simulink model "Microgrid_LCTLM_server"  (R2025b)
settings: Solver=ode3  StartTime=0.0  StopTime=1  FixedStep=params.sampleTime  RelTol=1e-3
InitFcn:
  | unitlmModelFile = get_param(bdroot, 'FileName');
  | if ~isempty(unitlmModelFile), addpath(fileparts(unitlmModelFile)); end
  | initialise_optimised_tlm_interface();
  | clear unitlmModelFile
StartFcn:
  | unitlmModelFile = get_param(bdroot, 'FileName'); if ~isempty(unitlmModelFile), addpath(fileparts(unitlmModelFile)); end; try, if exist('unitlm_timing_probe', 'file') == 2, unitlm_timing_probe('start', 'server', bdroot); else, warning('uniTLM:TimingProbeNotFound', 'unitlm_timing_probe.m not found on MATLAB path; timing probe disabled.'); end; catch unitlmTimingError, warning('uniTLM:TimingProbeFailed', 'unitlm_timing_probe failed: %s', unitlmTimingError.message); end; clear unitlmModelFile
StopFcn:
  | unitlmModelFile = get_param(bdroot, 'FileName'); if ~isempty(unitlmModelFile), addpath(fileparts(unitlmModelFile)); end; try, if exist('unitlm_timing_probe', 'file') == 2, unitlm_timing_probe('stop', 'server', bdroot); else, warning('uniTLM:TimingProbeNotFound', 'unitlm_timing_probe.m not found on MATLAB path; timing probe disabled.'); end; catch unitlmTimingError, warning('uniTLM:TimingProbeFailed', 'unitlm_timing_probe failed: %s', unitlmTimingError.message); end; clear unitlmModelFile
  | %% StopFcn: save TLM server-side results
  | 
  | modelName = bdroot;
  | modelFile = get_param(modelName, 'FileName');
  | 
  | if isempty(modelFile)
  |     modelDir = pwd;
  | else
  |     modelDir = fileparts(modelFile);
  | end
  | 
  | resultDir = fullfile(modelDir, 'result');
  | 
  | if ~exist(resultDir, 'dir')
  |     mkdir(resultDir);
  | end
  | 
  | % Server-side workspace variables
  | variableNames = {
  |     'server_voltage'
  |     'server_current'
  |     'server_PQ'
  | };
  | 
  | serverTLMData = struct();
  | 
  | for k = 1:numel(variableNames)
  | 
  |     originalName = variableNames{k};
  |     saveName = [originalName, '_TLM'];
  | 
  |     if evalin('base', sprintf('exist(''%s'', ''var'')', originalName))
  |         serverTLMData.(saveName) = evalin('base', originalName);
  |     else
  |         warning( ...
  |             'StopFcn:MissingVariable', ...
  |             'Variable "%s" was not found in the base workspace.', ...
  |             originalName);
  |     end
  | end
  | 
  | % Save to result/server_TLM.mat
  | saveFile = fullfile(resultDir, 'server_TLM.mat');
  | save(saveFile, '-struct', 'serverTLMData');
  | 
  | fprintf('TLM server-side results saved to:\n%s\n', saveFile);
values from neighbouring files (symbols this model uses):
  Cf = Cf_pu*Cb    [initialize_unitlm_microgrid.m]
  f = logspace(log10(fMin), log10(fMax), nFrequency).'    [fit_non_heaviside_line_rational.m]    (also in initialize_unitlm_microgrid.m = 50)
  fsw1 = 10e3    (= 10000)    [initialize_unitlm_microgrid.m]
  hr_lp_a = interface.hr_lp_a    [initialise_optimised_tlm_interface.m]
  hr_lp_b = interface.hr_lp_b    [initialise_optimised_tlm_interface.m]
  Ip = 2*P/(3*Vp)    [initialize_unitlm_microgrid.m]
  L1 = L1_pu*Lb    [initialize_unitlm_microgrid.m]
  L2 = L2_pu*Lb    [initialize_unitlm_microgrid.m]
  L3 = L3_pu*Lb    [initialize_unitlm_microgrid.m]
  L4 = L4_pu*Lb    [initialize_unitlm_microgrid.m]
  L_leakageinductance_1 = windingInductance(primaryWindingIndex)    [initialise_optimised_tlm_interface.m]
  L_magnetisation_1 = transformer.LmPu*primaryZbase/omegaNominal    [initialise_optimised_tlm_interface.m]
  L_remain_server = interface.L_remain_server    [initialise_optimised_tlm_interface.m]
  Lc = Lc_pu*Lb    [initialize_unitlm_microgrid.m]
  Lf2 = Lf2_pu*Lb    [initialize_unitlm_microgrid.m]
  line_aHr = interface.line_aHr    [initialise_optimised_tlm_interface.m]    (also in initialize_unitlm_microgrid.m = real(line_aHr))
  line_aZc = interface.line_aZc    [initialise_optimised_tlm_interface.m]    (also in initialize_unitlm_microgrid.m = real(line_aZc))
  line_bHr = interface.line_bHr    [initialise_optimised_tlm_interface.m]    (also in initialize_unitlm_microgrid.m = real(line_bHr))
  line_bZc = interface.line_bZc    [initialise_optimised_tlm_interface.m]    (also in initialize_unitlm_microgrid.m = real(line_bZc))
  P = 5e6    (= 5000000)    [initialize_unitlm_microgrid.m]
  params = varargin{1}    [Client_co.m]    (also in Client_co_TLM.m; Server_co.m; Server_co_TLM.m; initialise_optimised_tlm_interface.m = config.cosimParams)
  R1 = R1_pu*Zb    [initialize_unitlm_microgrid.m]
  R2 = R2_pu*Zb    [initialize_unitlm_microgrid.m]
  R3 = R3_pu*Zb    [initialize_unitlm_microgrid.m]
  R4 = R4_pu*Zb    [initialize_unitlm_microgrid.m]
  R_copperloss_1 = windingResistance(primaryWindingIndex)    [initialise_optimised_tlm_interface.m]
  R_coreloss_1 = transformer.RmPu*primaryZbase    [initialise_optimised_tlm_interface.m]
  R_remain_server = interface.R_remain_server    [initialise_optimised_tlm_interface.m]
  Rbreaker = Rbreaker_pu*Zb    [initialize_unitlm_microgrid.m]
  Rdamp = Rf    [initialize_unitlm_microgrid.m]
  Rf = Rf_pu*Zb    [initialize_unitlm_microgrid.m]
  Rload1 = Vp/Ip    [initialize_unitlm_microgrid.m]
  Rload2 = Vp/Ip    [initialize_unitlm_microgrid.m]
  Rload3 = Vp/Ip    [initialize_unitlm_microgrid.m]
  Rv_pu = 0.1    [initialize_unitlm_microgrid.m]
  Sxfmr = 6.3e6    (= 6300000)    [initialize_unitlm_microgrid.m]
  Vac = sqrt(2)*Vline/sqrt(3)    [initialize_unitlm_microgrid.m]
  Vhv = 66e3    (= 66000)    [initialize_unitlm_microgrid.m]
  Vline = 690    [initialize_unitlm_microgrid.m]
  Vp = Vac    [initialize_unitlm_microgrid.m]
  Wb = 2*pi*f    (= 314.159265359)    [initialize_unitlm_microgrid.m]
  Xv_pu = 0.3    [initialize_unitlm_microgrid.m]
  Zc_base_L = interface.Zc_base_L    [initialise_optimised_tlm_interface.m]
  Zc_base_R = interface.Zc_base_R    [initialise_optimised_tlm_interface.m]
undefined symbols (not defined in the file or in its folder): DiscIntNeverNeededParam, DPL, dspblkCoreblockFVToolHelper, gcbh, Lline1
libraries: spsThreePhaseSeriesRLCBranchLib x18, spsControlledVoltageSourceLib x12, spsThreePhaseVIMeasurementLib x7, spsabctodq0Lib x6, simulink x4, slpidlib x4, spsThreePhaseBreakerLib x4, SimplusGT x3, spsThreePhaseTransformerTwoWindingsLib x3, spsPower3phInstantaneousLib x2, spsdq0toabcLib x2, spsDistributedParametersLineLib x1
(part 3 of 4)

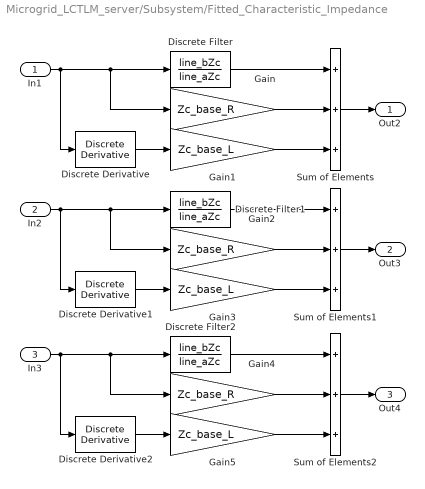
== system Microgrid_LCTLM_server/Subsystem/Fitted_Characteristic_Impedance ==
  In1 : Inport
  In2 : Inport  Port=2
  In3 : Inport  Port=3
  Discrete Derivative : simulink/Discrete/Discrete Derivative  gainval=1.0  ICPrevScaledInput=0.0  OutMin=[]  OutMax=[]  OutDataType=fixdt(1, 16)  OutScaling=2^-10  DoSatur=off
  Discrete Derivative1 : simulink/Discrete/Discrete Derivative  gainval=1.0  ICPrevScaledInput=0.0  OutMin=[]  OutMax=[]  OutDataType=fixdt(1, 16)  OutScaling=2^-10  DoSatur=off
  Discrete Derivative2 : simulink/Discrete/Discrete Derivative  gainval=1.0  ICPrevScaledInput=0.0  OutMin=[]  OutMax=[]  OutDataType=fixdt(1, 16)  OutScaling=2^-10  DoSatur=off
  Discrete Filter : DiscreteFilter  LoadFcn=dspblkCoreblockFVToolHelper(gcbh,'load');  Numerator=line_bZc  Denominator=line_aZc
      settings: CopyFcn=dspblkCoreblockFVToolHelper(gcbh,'copy');  DeleteFcn=dspblkCoreblockFVToolHelper(gcbh,'close');  ModelCloseFcn=dspblkCoreblockFVToolHelper(gcbh,'close');  PreSaveFcn=dspblkCoreblockFVToolHelper(gcbh,'presave');  PostSaveFcn=dspblkCoreblockFVToolHelper(gcbh,'postsave');  CloseFcn=dspblkCoreblockFVToolHelper(gcbh,'close');
  Discrete Filter1 : DiscreteFilter  LoadFcn=dspblkCoreblockFVToolHelper(gcbh,'load');  Numerator=line_bZc  Denominator=line_aZc
      settings: CopyFcn=dspblkCoreblockFVToolHelper(gcbh,'copy');  DeleteFcn=dspblkCoreblockFVToolHelper(gcbh,'close');  ModelCloseFcn=dspblkCoreblockFVToolHelper(gcbh,'close');  PreSaveFcn=dspblkCoreblockFVToolHelper(gcbh,'presave');  PostSaveFcn=dspblkCoreblockFVToolHelper(gcbh,'postsave');  CloseFcn=dspblkCoreblockFVToolHelper(gcbh,'close');
  Discrete Filter2 : DiscreteFilter  LoadFcn=dspblkCoreblockFVToolHelper(gcbh,'load');  Numerator=line_bZc  Denominator=line_aZc
      settings: CopyFcn=dspblkCoreblockFVToolHelper(gcbh,'copy');  DeleteFcn=dspblkCoreblockFVToolHelper(gcbh,'close');  ModelCloseFcn=dspblkCoreblockFVToolHelper(gcbh,'close');  PreSaveFcn=dspblkCoreblockFVToolHelper(gcbh,'presave');  PostSaveFcn=dspblkCoreblockFVToolHelper(gcbh,'postsave');  CloseFcn=dspblkCoreblockFVToolHelper(gcbh,'close');
  Gain : Gain  Gain=Zc_base_R
  Gain1 : Gain  Gain=Zc_base_L
  Gain2 : Gain  Gain=Zc_base_R
  Gain3 : Gain  Gain=Zc_base_L
  Gain4 : Gain  Gain=Zc_base_R
  Gain5 : Gain  Gain=Zc_base_L
  Sum of Elements : Sum  Inputs=+++
  Sum of Elements1 : Sum  Inputs=+++
  Sum of Elements2 : Sum  Inputs=+++
  Out2 : Outport
  Out3 : Outport  Port=2
  Out4 : Outport  Port=3
  wires:
  In1/1 -> Gain/1, Discrete Filter/1, Discrete Derivative/1
  Discrete Derivative/1 -> Gain1/1
  Gain/1 -> Sum of Elements/2
  Gain1/1 -> Sum of Elements/3
  Discrete Filter/1 -> Sum of Elements/1
  Sum of Elements/1 -> Out2/1
  Gain2/1 -> Sum of Elements1/2
  Discrete Filter1/1 -> Sum of Elements1/1
  Sum of Elements1/1 -> Out3/1
  Discrete Derivative1/1 -> Gain3/1
  Gain3/1 -> Sum of Elements1/3
  In2/1 -> Gain2/1, Discrete Filter1/1, Discrete Derivative1/1
  Gain5/1 -> Sum of Elements2/3
  Discrete Derivative2/1 -> Gain5/1
  Discrete Filter2/1 -> Sum of Elements2/1
  Gain4/1 -> Sum of Elements2/2
  Sum of Elements2/1 -> Out4/1
  In3/1 -> Gain4/1, Discrete Filter2/1, Discrete Derivative2/1

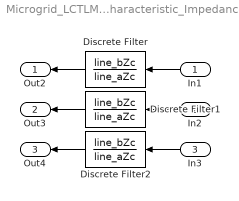
== system Microgrid_LCTLM_server/Subsystem/Fitted_Characteristic_Impedance1 ==
  In1 : Inport
  In2 : Inport  Port=2
  In3 : Inport  Port=3
  Discrete Filter : DiscreteFilter  LoadFcn=dspblkCoreblockFVToolHelper(gcbh,'load');  Numerator=line_bZc  Denominator=line_aZc
      settings: CopyFcn=dspblkCoreblockFVToolHelper(gcbh,'copy');  DeleteFcn=dspblkCoreblockFVToolHelper(gcbh,'close');  ModelCloseFcn=dspblkCoreblockFVToolHelper(gcbh,'close');  PreSaveFcn=dspblkCoreblockFVToolHelper(gcbh,'presave');  PostSaveFcn=dspblkCoreblockFVToolHelper(gcbh,'postsave');  CloseFcn=dspblkCoreblockFVToolHelper(gcbh,'close');
  Discrete Filter1 : DiscreteFilter  LoadFcn=dspblkCoreblockFVToolHelper(gcbh,'load');  Numerator=line_bZc  Denominator=line_aZc
      settings: CopyFcn=dspblkCoreblockFVToolHelper(gcbh,'copy');  DeleteFcn=dspblkCoreblockFVToolHelper(gcbh,'close');  ModelCloseFcn=dspblkCoreblockFVToolHelper(gcbh,'close');  PreSaveFcn=dspblkCoreblockFVToolHelper(gcbh,'presave');  PostSaveFcn=dspblkCoreblockFVToolHelper(gcbh,'postsave');  CloseFcn=dspblkCoreblockFVToolHelper(gcbh,'close');
  Discrete Filter2 : DiscreteFilter  LoadFcn=dspblkCoreblockFVToolHelper(gcbh,'load');  Numerator=line_bZc  Denominator=line_aZc
      settings: CopyFcn=dspblkCoreblockFVToolHelper(gcbh,'copy');  DeleteFcn=dspblkCoreblockFVToolHelper(gcbh,'close');  ModelCloseFcn=dspblkCoreblockFVToolHelper(gcbh,'close');  PreSaveFcn=dspblkCoreblockFVToolHelper(gcbh,'presave');  PostSaveFcn=dspblkCoreblockFVToolHelper(gcbh,'postsave');  CloseFcn=dspblkCoreblockFVToolHelper(gcbh,'close');
  Out2 : Outport
  Out3 : Outport  Port=2
  Out4 : Outport  Port=3
  wires:
  In1/1 -> Discrete Filter/1
  In2/1 -> Discrete Filter1/1
  Discrete Filter1/1 -> Out3/1
  Discrete Filter2/1 -> Out4/1
  In3/1 -> Discrete Filter2/1
  Discrete Filter/1 -> Out2/1

== system Microgrid_LCTLM_server/Subsystem/Grid1 ==
  Controlled Voltage Source1 : spsControlledVoltageSourceLib/Controlled Voltage Source  Initialize=on  Source_Type=AC  Amplitude=0  Phase=0  Frequency=0  Measurements=None
  Controlled Voltage Source2 : spsControlledVoltageSourceLib/Controlled Voltage Source  Initialize=on  Source_Type=AC  Amplitude=0  Phase=0  Frequency=0  Measurements=None
  Controlled Voltage Source6 : spsControlledVoltageSourceLib/Controlled Voltage Source  Initialize=on  Source_Type=AC  Amplitude=0  Phase=0  Frequency=0  Measurements=None
  Subsystem20 : Subsystem
  a : PMIOPort  Side=Left
  b : PMIOPort  Port=2  Side=Left
  c : PMIOPort  Port=3  Side=Left
  wires:
  Subsystem20/3(Ec) -> Controlled Voltage Source6/1
  Subsystem20/1(Ea) -> Controlled Voltage Source1/1
  Subsystem20/2(Eb) -> Controlled Voltage Source2/1
  connections:
  Controlled Voltage Source1/RConn1 -- a/RConn1
  Controlled Voltage Source6/RConn1 -- c/RConn1
  Controlled Voltage Source6/LConn1 -- Controlled Voltage Source2/LConn1 -- Controlled Voltage Source1/LConn1
  Controlled Voltage Source2/RConn1 -- b/RConn1

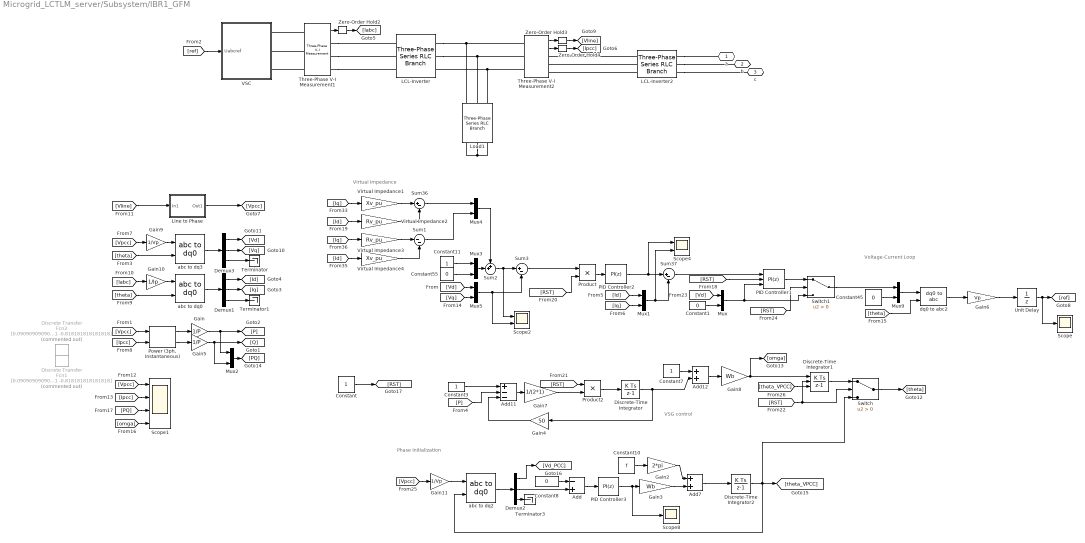
== system Microgrid_LCTLM_server/Subsystem/IBR1_GFM ==
  note: Voltage-Current Loop
  note: VSG control
  note: Virtual Impedance
  note: Phase Initialization
  Add : Sum  Inputs=-+
  Add11 : Sum  Inputs=+--
  Add12 : Sum
  Add7 : Sum
  Constant : Constant
  Constant{1,8,45,55} (4 alike) : Constant  Value=0
  Constant10 : Constant  Value=f
  Constant11 : Constant  SampleTime=-1
  Constant3 : Constant
  Constant7 : Constant
  Demux1 : Demux  Outputs=3
  Demux2 : Demux  Outputs=3
  Demux3 : Demux  Outputs=3
  Discrete Transfer Fcn1 : DiscreteTransferFcn  Commented=on  Numerator=[0.090909090909091 0.090909090909091]  Denominator=[1 -0.818181818181818]
  Discrete Transfer Fcn2 : DiscreteTransferFcn  Commented=on  Numerator=[0.090909090909091 0.090909090909091]  Denominator=[1 -0.818181818181818]
  Discrete-Time Integrator : DiscreteIntegrator  SampleTime=1/fsw1  ICPrevOutput=DiscIntNeverNeededParam  ICPrevScaledInput=DiscIntNeverNeededParam
  Discrete-Time Integrator1 : DiscreteIntegrator  ExternalReset=rising  InitialConditionSource=external  SampleTime=1/fsw1  ICPrevOutput=DiscIntNeverNeededParam  ICPrevScaledInput=DiscIntNeverNeededParam
  Discrete-Time Integrator2 : DiscreteIntegrator  SampleTime=1/fsw1  ICPrevOutput=DiscIntNeverNeededParam  ICPrevScaledInput=DiscIntNeverNeededParam
  Gain : Gain  Gain=1/P
  Gain10 : Gain  Gain=1/Ip
  Gain11 : Gain  Gain=1/Vp
  Gain2 : Gain  Gain=2*pi
  Gain3 : Gain  Gain=Wb
  Gain4 : Gain  Gain=50
  Gain5 : Gain  Gain=1/P
  Gain6 : Gain  Gain=Vp
  Gain7 : Gain  Gain=1/(2*1)
  Gain8 : Gain  Gain=Wb
  Gain9 : Gain  Gain=1/Vp
  LCL-Inverter : spsThreePhaseSeriesRLCBranchLib/Three-Phase Series RLC Branch  LConnTagsString=A|B|C  RConnTagsString=A|B|C  BranchType=RL  Resistance=Rf  Inductance=Lc  Capacitance=1e-6  Measurements=None
  LCL-Inverter2 : spsThreePhaseSeriesRLCBranchLib/Three-Phase Series RLC Branch  LConnTagsString=A|B|C  RConnTagsString=A|B|C  BranchType=RL  Resistance=Rf  Inductance=Lf2  Capacitance=1e-6  Measurements=None
  Line to Phase : Subsystem
  Load1 : spsThreePhaseSeriesRLCBranchLib/Three-Phase Series RLC Branch  LConnTagsString=A|B|C  RConnTagsString=A|B|C  BranchType=RC  Resistance=Rdamp  Inductance=1e-3  Capacitance=Cf  Measurements=None
  Mux{,1..5,9} (7 alike) : Mux  Inputs=2
  PID Controller1 : slpidlib/PID Controller  Controller=PI  Form=Parallel  TimeDomain=Discrete-time  UseExternalTs=off  SampleTime=1/fsw1  IntegratorMethod=Forward Euler  FilterMethod=Forward Euler  ControllerParametersSource=internal  P=0.5  I=100  UseKiTs=off  D=0  UseExternalDerivativeSource=off  N=100  UseFilter=on  TunerSelectOption=Transfer Function Based (PID Tuner App)  InitialConditionSource=external  InitialConditionForIntegrator=0  InitialConditionForFilter=0  DifferentiatorICPrevScaledInput=0  ExternalReset=rising  TrackingMode=off  Kt=1  LimitOutput=off  SatLimitsSource=internal  UpperSaturationLimit=inf  LowerSaturationLimit=-inf  LinearizeAsGain=on  AntiWindupMode=none  Kb=1  LimitIntegrator=off  UpperIntegratorSaturationLimit=inf  LowerIntegratorSaturationLimit=-inf  POutMin=[]  POutMax=[]  IOutMin=[]  IOutMax=[]  DOutMin=[]  DOutMax=[]  NOutMin=[]  NOutMax=[]  SumOutMin=[]  SumOutMax=[]  SaturationOutMin=[]  SaturationOutMax=[]  PParamMin=[]  PParamMax=[]  IParamMin=[]  IParamMax=[]  DParamMin=[]  DParamMax=[]  NParamMin=[]  NParamMax=[]  KbParamMin=[]  KbParamMax=[]  KtParamMin=[]  KtParamMax=[]  KbOutMin=[]  KbOutMax=[]  KtOutMin=[]  KtOutMax=[]  IntegratorOutMin=[]  IntegratorOutMax=[]  FilterOutMin=[]  FilterOutMax=[]  SumI1OutMin=[]  SumI1OutMax=[]  SumI2OutMin=[]  SumI2OutMax=[]  SumI3OutMin=[]  SumI3OutMax=[]  SumI4OutMin=[]  SumI4OutMax=[]  SumDOutMin=[]  SumDOutMax=[]  DifferentiatorOutMin=[]  DifferentiatorOutMax=[]  FilterDiffOutCoefMin=[]  FilterDiffOutCoefMax=[]  ReciprocalOutMin=[]  ReciprocalOutMax=[]  SumDenOutMin=[]  SumDenOutMax=[]  SumNumOutMin=[]  SumNumOutMax=[]  DivideOutMin=[]  DivideOutMax=[]  UdiffTsProdOutMin=[]  UdiffTsProdOutMax=[]  NTsProdOutMin=[]  NTsProdOutMax=[]  UintegralTsProdOutMin=[]  UintegralTsProdOutMax=[]  UngainTsProdOutMin=[]  UngainTsProdOutMax=[]  ClampingZeroOutDataTypeStr=Inherit: Inherit via back propagation  ClampingZeroOutMin=[]  ClampingZeroOutMax=[]  FilterDenConstantOutDataTypeStr=Inherit: Inherit via back propagation  FilterDenConstantOutMin=[]  FilterDenConstantOutMax=[]  PCopyOutDataTypeStr=Inherit: Inherit via back propagation  PCopyOutMin=[]  PCopyOutMax=[]  NCopyOutDataTypeStr=Inherit: Inherit via back propagation  NCopyOutMin=[]  NCopyOutMax=[]  IntegratorContinuousStateAttributes=''  IntegratorStateMustResolveToSignalObject=off  IntegratorRTWStateStorageClass=Auto  FilterContinuousStateAttributes=''  FilterStateMustResolveToSignalObject=off  FilterRTWStateStorageClass=Auto  ParallelPVariant=InternalParameters  IdealPVariant=Disabled  IVariant=InternalParameters  DVariant=Disabled  IntegratorVariant=Discrete  SatVariant=Disabled  AWVariant=Passthrough  PCopyVariant=Disabled  TRVariant=Disabled  FdbkBlocksVariant=Forward  IdealPFdbkVariant=Disabled  SatFdbkVariant=Disabled  DerivativeFilterVariant=Disabled  NVariant=Disabled  NCopyVariant=Disabled_SignalSpec  FilterICVariant=Disabled  IntegratorICVariant=ExternalICs  ExternalResetVariant=ExternalReset  TRSumVariant=Passthrough  SumFdbkVariant=Disabled  SumVariant=Sum_PI  TsampFilterVariant=InternalTs  TsampNgainVariant=Passthrough  TsampIntegralVariant=Disabled_SignalSpec  ExternalSaturationOutDataTypeStr=Inherit: Same as second input  DerivativeSourceVariant=Disabled  PreIntVariant=InternalPreInt
  PID Controller2 : slpidlib/PID Controller  Controller=PI  Form=Parallel  TimeDomain=Discrete-time  UseExternalTs=off  SampleTime=1/fsw1  IntegratorMethod=Forward Euler  FilterMethod=Forward Euler  ControllerParametersSource=internal  P=0.2  I=500  UseKiTs=off  D=0  UseExternalDerivativeSource=off  N=100  UseFilter=on  TunerSelectOption=Transfer Function Based (PID Tuner App)  InitialConditionSource=internal  InitialConditionForIntegrator=0  InitialConditionForFilter=0  DifferentiatorICPrevScaledInput=0  ExternalReset=none  TrackingMode=off  Kt=1  LimitOutput=off  SatLimitsSource=internal  UpperSaturationLimit=inf  LowerSaturationLimit=-inf  LinearizeAsGain=on  AntiWindupMode=none  Kb=1  LimitIntegrator=off  UpperIntegratorSaturationLimit=inf  LowerIntegratorSaturationLimit=-inf  POutMin=[]  POutMax=[]  IOutMin=[]  IOutMax=[]  DOutMin=[]  DOutMax=[]  NOutMin=[]  NOutMax=[]  SumOutMin=[]  SumOutMax=[]  SaturationOutMin=[]  SaturationOutMax=[]  PParamMin=[]  PParamMax=[]  IParamMin=[]  IParamMax=[]  DParamMin=[]  DParamMax=[]  NParamMin=[]  NParamMax=[]  KbParamMin=[]  KbParamMax=[]  KtParamMin=[]  KtParamMax=[]  KbOutMin=[]  KbOutMax=[]  KtOutMin=[]  KtOutMax=[]  IntegratorOutMin=[]  IntegratorOutMax=[]  FilterOutMin=[]  FilterOutMax=[]  SumI1OutMin=[]  SumI1OutMax=[]  SumI2OutMin=[]  SumI2OutMax=[]  SumI3OutMin=[]  SumI3OutMax=[]  SumI4OutMin=[]  SumI4OutMax=[]  SumDOutMin=[]  SumDOutMax=[]  DifferentiatorOutMin=[]  DifferentiatorOutMax=[]  FilterDiffOutCoefMin=[]  FilterDiffOutCoefMax=[]  ReciprocalOutMin=[]  ReciprocalOutMax=[]  SumDenOutMin=[]  SumDenOutMax=[]  SumNumOutMin=[]  SumNumOutMax=[]  DivideOutMin=[]  DivideOutMax=[]  UdiffTsProdOutMin=[]  UdiffTsProdOutMax=[]  NTsProdOutMin=[]  NTsProdOutMax=[]  UintegralTsProdOutMin=[]  UintegralTsProdOutMax=[]  UngainTsProdOutMin=[]  UngainTsProdOutMax=[]  ClampingZeroOutDataTypeStr=Inherit: Inherit via back propagation  ClampingZeroOutMin=[]  ClampingZeroOutMax=[]  FilterDenConstantOutDataTypeStr=Inherit: Inherit via back propagation  FilterDenConstantOutMin=[]  FilterDenConstantOutMax=[]  PCopyOutDataTypeStr=Inherit: Inherit via back propagation  PCopyOutMin=[]  PCopyOutMax=[]  NCopyOutDataTypeStr=Inherit: Inherit via back propagation  NCopyOutMin=[]  NCopyOutMax=[]  IntegratorContinuousStateAttributes=''  IntegratorStateMustResolveToSignalObject=off  IntegratorRTWStateStorageClass=Auto  FilterContinuousStateAttributes=''  FilterStateMustResolveToSignalObject=off  FilterRTWStateStorageClass=Auto  ParallelPVariant=InternalParameters  IdealPVariant=Disabled  IVariant=InternalParameters  DVariant=Disabled  IntegratorVariant=Discrete  SatVariant=Disabled  AWVariant=Passthrough  PCopyVariant=Disabled  TRVariant=Disabled  FdbkBlocksVariant=Forward  IdealPFdbkVariant=Disabled  SatFdbkVariant=Disabled  DerivativeFilterVariant=Disabled  NVariant=Disabled  NCopyVariant=Disabled_SignalSpec  FilterICVariant=Disabled  IntegratorICVariant=InternalICs  ExternalResetVariant=Disabled  TRSumVariant=Passthrough  SumFdbkVariant=Disabled  SumVariant=Sum_PI  TsampFilterVariant=InternalTs  TsampNgainVariant=Passthrough  TsampIntegralVariant=Disabled_SignalSpec  ExternalSaturationOutDataTypeStr=Inherit: Same as second input  DerivativeSourceVariant=Disabled  PreIntVariant=InternalPreInt
  PID Controller3 : slpidlib/PID Controller  Controller=PI  Form=Parallel  TimeDomain=Discrete-time  UseExternalTs=off  SampleTime=1/fsw1  IntegratorMethod=Forward Euler  FilterMethod=Forward Euler  ControllerParametersSource=internal  P=2  I=5  UseKiTs=off  D=0  UseExternalDerivativeSource=off  N=100  UseFilter=on  TunerSelectOption=Transfer Function Based (PID Tuner App)  InitialConditionSource=internal  InitialConditionForIntegrator=0  InitialConditionForFilter=0  DifferentiatorICPrevScaledInput=0  ExternalReset=none  TrackingMode=off  Kt=1  LimitOutput=off  SatLimitsSource=internal  UpperSaturationLimit=inf  LowerSaturationLimit=-inf  LinearizeAsGain=on  AntiWindupMode=none  Kb=1  LimitIntegrator=off  UpperIntegratorSaturationLimit=inf  LowerIntegratorSaturationLimit=-inf  POutMin=[]  POutMax=[]  IOutMin=[]  IOutMax=[]  DOutMin=[]  DOutMax=[]  NOutMin=[]  NOutMax=[]  SumOutMin=[]  SumOutMax=[]  SaturationOutMin=[]  SaturationOutMax=[]  PParamMin=[]  PParamMax=[]  IParamMin=[]  IParamMax=[]  DParamMin=[]  DParamMax=[]  NParamMin=[]  NParamMax=[]  KbParamMin=[]  KbParamMax=[]  KtParamMin=[]  KtParamMax=[]  KbOutMin=[]  KbOutMax=[]  KtOutMin=[]  KtOutMax=[]  IntegratorOutMin=[]  IntegratorOutMax=[]  FilterOutMin=[]  FilterOutMax=[]  SumI1OutMin=[]  SumI1OutMax=[]  SumI2OutMin=[]  SumI2OutMax=[]  SumI3OutMin=[]  SumI3OutMax=[]  SumI4OutMin=[]  SumI4OutMax=[]  SumDOutMin=[]  SumDOutMax=[]  DifferentiatorOutMin=[]  DifferentiatorOutMax=[]  FilterDiffOutCoefMin=[]  FilterDiffOutCoefMax=[]  ReciprocalOutMin=[]  ReciprocalOutMax=[]  SumDenOutMin=[]  SumDenOutMax=[]  SumNumOutMin=[]  SumNumOutMax=[]  DivideOutMin=[]  DivideOutMax=[]  UdiffTsProdOutMin=[]  UdiffTsProdOutMax=[]  NTsProdOutMin=[]  NTsProdOutMax=[]  UintegralTsProdOutMin=[]  UintegralTsProdOutMax=[]  UngainTsProdOutMin=[]  UngainTsProdOutMax=[]  ClampingZeroOutDataTypeStr=Inherit: Inherit via back propagation  ClampingZeroOutMin=[]  ClampingZeroOutMax=[]  FilterDenConstantOutDataTypeStr=Inherit: Inherit via back propagation  FilterDenConstantOutMin=[]  FilterDenConstantOutMax=[]  PCopyOutDataTypeStr=Inherit: Inherit via back propagation  PCopyOutMin=[]  PCopyOutMax=[]  NCopyOutDataTypeStr=Inherit: Inherit via back propagation  NCopyOutMin=[]  NCopyOutMax=[]  IntegratorContinuousStateAttributes=''  IntegratorStateMustResolveToSignalObject=off  IntegratorRTWStateStorageClass=Auto  FilterContinuousStateAttributes=''  FilterStateMustResolveToSignalObject=off  FilterRTWStateStorageClass=Auto  ParallelPVariant=InternalParameters  IdealPVariant=Disabled  IVariant=InternalParameters  DVariant=Disabled  IntegratorVariant=Discrete  SatVariant=Disabled  AWVariant=Passthrough  PCopyVariant=Disabled  TRVariant=Disabled  FdbkBlocksVariant=Forward  IdealPFdbkVariant=Disabled  SatFdbkVariant=Disabled  DerivativeFilterVariant=Disabled  NVariant=Disabled  NCopyVariant=Disabled_SignalSpec  FilterICVariant=Disabled  IntegratorICVariant=InternalICs  ExternalResetVariant=Disabled  TRSumVariant=Passthrough  SumFdbkVariant=Disabled  SumVariant=Sum_PI  TsampFilterVariant=InternalTs  TsampNgainVariant=Passthrough  TsampIntegralVariant=Disabled_SignalSpec  ExternalSaturationOutDataTypeStr=Inherit: Same as second input  DerivativeSourceVariant=Disabled  PreIntVariant=InternalPreInt
  "Power (3ph, Instantaneous)" : spsPower3phInstantaneousLib/Power (3ph, Instantaneous)
  Product : Product
  Product2 : Product
  Scope : Scope
      settings: ActiveDisplayYMinimum=-1487.20088  ActiveDisplayYMaximum=1156.37442  DataLoggingVariableName=ScopeData2
  Scope1 : Scope  NumInputPorts=4
      settings: ActiveDisplayYMinimum=-459.19644  ActiveDisplayYMaximum=463.11203  DataLoggingVariableName=ScopeData4
  Scope2 : Scope  NumInputPorts=2
      settings: ActiveDisplayYMinimum=-0.48353  ActiveDisplayYMaximum=1.26771
  Scope4 : Scope  NumInputPorts=2
      settings: ActiveDisplayYMinimum=-1.96338  ActiveDisplayYMaximum=2.79764  DataLoggingVariableName=ScopeData3
  Scope8 : Scope
      settings: ActiveDisplayYMinimum=-0.17841  ActiveDisplayYMaximum=0.07598  DataLoggingVariableName=ScopeData4
  Sum1 : Sum  Inputs=|--
  Sum2 : Sum  Inputs=++|
  Sum3 : Sum  Inputs=|+-
  Sum36 : Sum  Inputs=|+-
  Sum37 : Sum  Inputs=|+-
  Switch : Switch  Criteria=u2 > Threshold  SaturateOnIntegerOverflow=off  InputSameDT=off
  Switch1 : Switch  Criteria=u2 > Threshold  SaturateOnIntegerOverflow=off  InputSameDT=off
  Terminator : Terminator
  Terminator1 : Terminator
  Terminator3 : Terminator
  Three-Phase V-I Measurement1 : spsThreePhaseVIMeasurementLib/Three-Phase V-I Measurement  VoltageMeasurement=no  SetLabelV=off  LabelV=Vabc  Vpu=off  VpuLL=off  CurrentMeasurement=yes  SetLabelI=off  LabelI=Iabc  Ipu=off  Pbase=100e6  Vbase=500e3  OutputType=Complex  PhasorSimulation=off  PSBequivalent=0
  Three-Phase V-I Measurement2 : spsThreePhaseVIMeasurementLib/Three-Phase V-I Measurement  VoltageMeasurement=phase-to-phase  SetLabelV=off  LabelV=Vabc  Vpu=off  VpuLL=off  CurrentMeasurement=yes  SetLabelI=off  LabelI=Iabc  Ipu=off  Pbase=100e6  Vbase=500e3  OutputType=Complex  PhasorSimulation=off  PSBequivalent=0
  Unit Delay : UnitDelay  SampleTime=1/fsw1
  VSC : Subsystem
  Virtual Impedance1 : Gain  Gain=Xv_pu
  Virtual Impedance2 : Gain  Gain=Rv_pu
  Virtual Impedance3 : Gain  Gain=Rv_pu
  Virtual Impedance4 : Gain  Gain=Xv_pu
  Zero-Order Hold2 : ZeroOrderHold  SampleTime=1/fsw1
  Zero-Order Hold3 : ZeroOrderHold  SampleTime=1/fsw1
  Zero-Order Hold4 : ZeroOrderHold  SampleTime=1/fsw1
  abc to dq0 : spsabctodq0Lib/abc to dq0  Alignment=90 degrees behind phase A axis
  abc to dq2 : spsabctodq0Lib/abc to dq0  Alignment=90 degrees behind phase A axis
  abc to dq3 : spsabctodq0Lib/abc to dq0  Alignment=90 degrees behind phase A axis
  dq0 to abc2 : spsdq0toabcLib/dq0 to abc  Alignment=90 degrees behind phase A axis
  a : PMIOPort  Side=Right
  b : PMIOPort  Port=2  Side=Right
  c : PMIOPort  Port=3  Side=Right
  wires:
  Mux2/1 -> [PQ]
  [omga] -> Scope1/4
  [PQ] -> Scope1/3
  "Power (3ph, Instantaneous)"/1 -> Gain/1
  "Power (3ph, Instantaneous)"/2 -> Gain5/1
  [Ipcc] -> "Power (3ph, Instantaneous)"/2
  [Vpcc] -> "Power (3ph, Instantaneous)"/1
  [ref] -> VSC/1(Uabcref)
  Demux3/2 -> [Vq]
  Constant55/1 -> Mux3/2
  Mux9/1 -> dq0 to abc2/1
  [Vq] -> Mux5/2
  Add12/1 -> Gain8/1
  Constant3/1 -> Add11/1
  Mux3/1 -> Sum2/2
  Discrete-Time Integrator/1 -> Add12/2, Gain4/1
  Gain4/1 -> Add11/3
  [Vpcc] -> Gain9/1
  [Iq] -> Mux1/2
  Demux3/3 -> Terminator/1
  Constant45/1 -> Mux9/2
  Add11/1 -> Gain7/1
  [theta] -> abc to dq3/2
  [P] -> Add11/2
  dq0 to abc2/1 -> Gain6/1
  [Id] -> Mux1/1
  [theta] -> abc to dq0/2
  Unit Delay/1 -> Scope/1, [ref]
  Constant11/1 -> Mux3/1
  [Vd] -> Mux5/1
  PID Controller2/1 -> Scope4/1, Sum37/1
  Mux1/1 -> Scope4/2, Sum37/2
  Demux3/1 -> [Vd]
  Gain6/1 -> Unit Delay/1
  Gain10/1 -> abc to dq0/1
  Mux5/1 -> Sum3/2, Scope2/2
  abc to dq3/1 -> Demux3/1
  Constant7/1 -> Add12/1
  [theta] -> dq0 to abc2/2
  Three-Phase V-I Measurement1/1 -> Zero-Order Hold2/1
  Zero-Order Hold2/1 -> [Iabc]
  Three-Phase V-I Measurement2/2 -> Zero-Order Hold4/1
  Three-Phase V-I Measurement2/1 -> Zero-Order Hold3/1
  Zero-Order Hold3/1 -> [Vline]
  Zero-Order Hold4/1 -> [Ipcc]
  Gain9/1 -> abc to dq3/1
  [Iabc] -> Gain10/1
  abc to dq0/1 -> Demux1/1
  Demux1/1 -> [Id]
  Demux1/3 -> Terminator1/1
  Demux1/2 -> [Iq]
  [Vline] -> Line to Phase/1(In1)
  Line to Phase/1(Out1) -> [Vpcc]
  [Vpcc] -> Scope1/1
  [Ipcc] -> Scope1/2
  Gain/1 -> Mux2/1, [P]
  Gain5/1 -> Mux2/2, [Q]
  [Iq] -> Virtual Impedance3/1
  [Id] -> Virtual Impedance4/1
  [Id] -> Virtual Impedance2/1
  Sum36/1 -> Mux4/1
  [Iq] -> Virtual Impedance1/1
  Virtual Impedance1/1 -> Sum36/1
  Sum1/1 -> Mux4/2
  Virtual Impedance2/1 -> Sum36/2
  Virtual Impedance4/1 -> Sum1/2
  Virtual Impedance3/1 -> Sum1/1
  Mux4/1 -> Sum2/1
  [RST] -> Product/2
  Product/1 -> PID Controller2/1
  [RST] -> PID Controller1/2
  Gain7/1 -> Product2/2
  Product2/1 -> Discrete-Time Integrator/1
  [RST] -> Product2/1
  [RST] -> Switch/2, Discrete-Time Integrator1/2
  PID Controller3/1 -> Scope8/1, Gain3/1
  Constant8/1 -> Add/1
  abc to dq2/1 -> Demux2/1
  Demux2/2 -> Add/2
  Demux2/3 -> Terminator3/1
  [Vpcc] -> Gain11/1
  Constant10/1 -> Gain2/1
  Add/1 -> PID Controller3/1
  Gain2/1 -> Add7/1
  Gain3/1 -> Add7/2
  Discrete-Time Integrator2/1 -> Switch/3, [theta_VPCC], abc to dq2/2
  Gain11/1 -> abc to dq2/1
  Add7/1 -> Discrete-Time Integrator2/1
  Constant1/1 -> Mux/2
  [Vd] -> Mux/1
  Mux/1 -> Switch1/3, PID Controller1/3
  Constant/1 -> [RST]
  Gain8/1 -> Discrete-Time Integrator1/1, [omga]
  [theta_VPCC] -> Discrete-Time Integrator1/3
  Discrete-Time Integrator1/1 -> Switch/1
  Switch/1 -> [theta]
  PID Controller1/1 -> Switch1/1
  Switch1/1 -> Mux9/1
  [RST] -> Switch1/2
  Sum37/1 -> PID Controller1/1
  Sum2/1 -> Scope2/1, Sum3/1
  Sum3/1 -> Product/1
  Demux2/1 -> [Vd_PCC]
  connections:
  LCL-Inverter2/RConn1 -- a/RConn1
  Three-Phase V-I Measurement1/RConn1 -- LCL-Inverter/LConn1
  Load1/LConn2 -- LCL-Inverter/RConn2 -- Three-Phase V-I Measurement2/LConn2
  Load1/LConn3 -- LCL-Inverter/RConn3 -- Three-Phase V-I Measurement2/LConn3
  Load1/LConn1 -- LCL-Inverter/RConn1 -- Three-Phase V-I Measurement2/LConn1
  Three-Phase V-I Measurement1/RConn2 -- LCL-Inverter/LConn2
  Three-Phase V-I Measurement1/RConn3 -- LCL-Inverter/LConn3
  LCL-Inverter2/RConn2 -- b/RConn1
  LCL-Inverter2/LConn1 -- Three-Phase V-I Measurement2/RConn1
  LCL-Inverter2/RConn3 -- c/RConn1
  Load1/RConn3 -- Load1/RConn2 -- Load1/RConn1
  Three-Phase V-I Measurement1/LConn1 -- VSC/RConn1
  Three-Phase V-I Measurement1/LConn2 -- VSC/RConn2
  Three-Phase V-I Measurement1/LConn3 -- VSC/RConn3
  LCL-Inverter2/LConn2 -- Three-Phase V-I Measurement2/RConn2
  LCL-Inverter2/LConn3 -- Three-Phase V-I Measurement2/RConn3

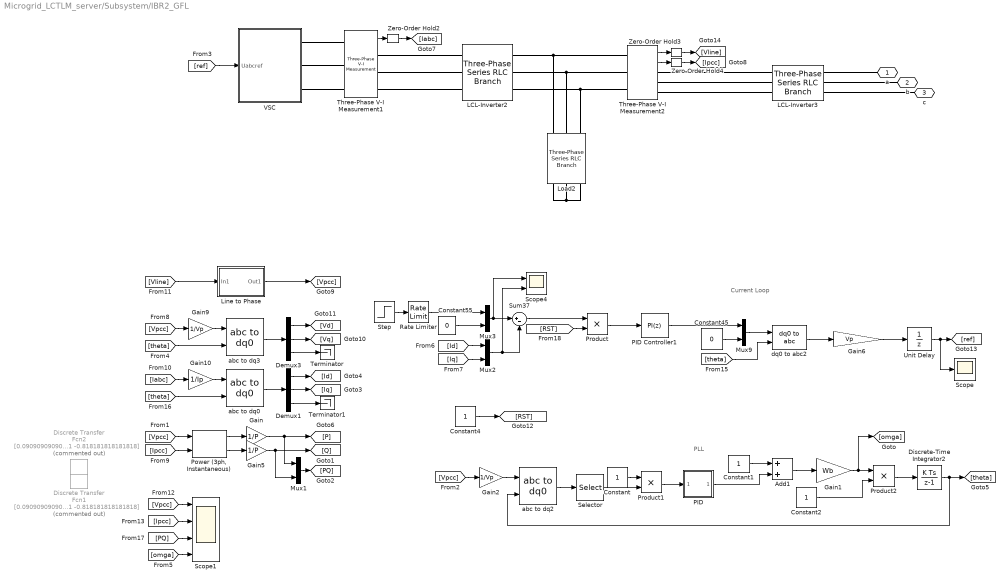
== system Microgrid_LCTLM_server/Subsystem/IBR2_GFL ==
  note: Current Loop
  note: PLL
  Add1 : Sum
  Constant{,1..2,4} (4 alike) : Constant
  Constant45 : Constant  Value=0
  Constant55 : Constant  Value=0
  Demux1 : Demux  Outputs=3
  Demux3 : Demux  Outputs=3
  Discrete Transfer Fcn1 : DiscreteTransferFcn  Commented=on  Numerator=[0.090909090909091 0.090909090909091]  Denominator=[1 -0.818181818181818]
  Discrete Transfer Fcn2 : DiscreteTransferFcn  Commented=on  Numerator=[0.090909090909091 0.090909090909091]  Denominator=[1 -0.818181818181818]
  Discrete-Time Integrator2 : DiscreteIntegrator  SampleTime=1/fsw1  ICPrevOutput=DiscIntNeverNeededParam  ICPrevScaledInput=DiscIntNeverNeededParam
  Gain : Gain  Gain=1/P
  Gain1 : Gain  Gain=Wb
  Gain10 : Gain  Gain=1/Ip
  Gain2 : Gain  Gain=1/Vp
  Gain5 : Gain  Gain=1/P
  Gain6 : Gain  Gain=Vp
  Gain9 : Gain  Gain=1/Vp
  LCL-Inverter2 : spsThreePhaseSeriesRLCBranchLib/Three-Phase Series RLC Branch  LConnTagsString=A|B|C  RConnTagsString=A|B|C  BranchType=RL  Resistance=Rf  Inductance=Lc  Capacitance=1e-6  Measurements=None
  LCL-Inverter3 : spsThreePhaseSeriesRLCBranchLib/Three-Phase Series RLC Branch  LConnTagsString=A|B|C  RConnTagsString=A|B|C  BranchType=RL  Resistance=Rf  Inductance=Lf2  Capacitance=1e-6  Measurements=None
  Line to Phase : Subsystem
  Load2 : spsThreePhaseSeriesRLCBranchLib/Three-Phase Series RLC Branch  LConnTagsString=A|B|C  RConnTagsString=A|B|C  BranchType=RC  Resistance=Rdamp  Inductance=1e-3  Capacitance=Cf  Measurements=None
  Mux{1..3,9} (4 alike) : Mux  Inputs=2
  PID : Subsystem
  PID Controller1 : slpidlib/PID Controller  Controller=PI  Form=Parallel  TimeDomain=Discrete-time  UseExternalTs=off  SampleTime=1/fsw1  IntegratorMethod=Forward Euler  FilterMethod=Forward Euler  ControllerParametersSource=internal  P=0.5  I=100  UseKiTs=off  D=0  UseExternalDerivativeSource=off  N=100  UseFilter=on  TunerSelectOption=Transfer Function Based (PID Tuner App)  InitialConditionSource=internal  InitialConditionForIntegrator=[1;0]  InitialConditionForFilter=0  DifferentiatorICPrevScaledInput=0  ExternalReset=none  TrackingMode=off  Kt=1  LimitOutput=off  SatLimitsSource=internal  UpperSaturationLimit=inf  LowerSaturationLimit=-inf  LinearizeAsGain=on  AntiWindupMode=none  Kb=1  LimitIntegrator=off  UpperIntegratorSaturationLimit=inf  LowerIntegratorSaturationLimit=-inf  POutMin=[]  POutMax=[]  IOutMin=[]  IOutMax=[]  DOutMin=[]  DOutMax=[]  NOutMin=[]  NOutMax=[]  SumOutMin=[]  SumOutMax=[]  SaturationOutMin=[]  SaturationOutMax=[]  PParamMin=[]  PParamMax=[]  IParamMin=[]  IParamMax=[]  DParamMin=[]  DParamMax=[]  NParamMin=[]  NParamMax=[]  KbParamMin=[]  KbParamMax=[]  KtParamMin=[]  KtParamMax=[]  KbOutMin=[]  KbOutMax=[]  KtOutMin=[]  KtOutMax=[]  IntegratorOutMin=[]  IntegratorOutMax=[]  FilterOutMin=[]  FilterOutMax=[]  SumI1OutMin=[]  SumI1OutMax=[]  SumI2OutMin=[]  SumI2OutMax=[]  SumI3OutMin=[]  SumI3OutMax=[]  SumI4OutMin=[]  SumI4OutMax=[]  SumDOutMin=[]  SumDOutMax=[]  DifferentiatorOutMin=[]  DifferentiatorOutMax=[]  FilterDiffOutCoefMin=[]  FilterDiffOutCoefMax=[]  ReciprocalOutMin=[]  ReciprocalOutMax=[]  SumDenOutMin=[]  SumDenOutMax=[]  SumNumOutMin=[]  SumNumOutMax=[]  DivideOutMin=[]  DivideOutMax=[]  UdiffTsProdOutMin=[]  UdiffTsProdOutMax=[]  NTsProdOutMin=[]  NTsProdOutMax=[]  UintegralTsProdOutMin=[]  UintegralTsProdOutMax=[]  UngainTsProdOutMin=[]  UngainTsProdOutMax=[]  ClampingZeroOutDataTypeStr=Inherit: Inherit via back propagation  ClampingZeroOutMin=[]  ClampingZeroOutMax=[]  FilterDenConstantOutDataTypeStr=Inherit: Inherit via back propagation  FilterDenConstantOutMin=[]  FilterDenConstantOutMax=[]  PCopyOutDataTypeStr=Inherit: Inherit via back propagation  PCopyOutMin=[]  PCopyOutMax=[]  NCopyOutDataTypeStr=Inherit: Inherit via back propagation  NCopyOutMin=[]  NCopyOutMax=[]  IntegratorContinuousStateAttributes=''  IntegratorStateMustResolveToSignalObject=off  IntegratorRTWStateStorageClass=Auto  FilterContinuousStateAttributes=''  FilterStateMustResolveToSignalObject=off  FilterRTWStateStorageClass=Auto  ParallelPVariant=InternalParameters  IdealPVariant=Disabled  IVariant=InternalParameters  DVariant=Disabled  IntegratorVariant=Discrete  SatVariant=Disabled  AWVariant=Passthrough  PCopyVariant=Disabled  TRVariant=Disabled  FdbkBlocksVariant=Forward  IdealPFdbkVariant=Disabled  SatFdbkVariant=Disabled  DerivativeFilterVariant=Disabled  NVariant=Disabled  NCopyVariant=Disabled_SignalSpec  FilterICVariant=Disabled  IntegratorICVariant=InternalICs  ExternalResetVariant=Disabled  TRSumVariant=Passthrough  SumFdbkVariant=Disabled  SumVariant=Sum_PI  TsampFilterVariant=InternalTs  TsampNgainVariant=Passthrough  TsampIntegralVariant=Disabled_SignalSpec  ExternalSaturationOutDataTypeStr=Inherit: Same as second input  DerivativeSourceVariant=Disabled  PreIntVariant=InternalPreInt
  "Power (3ph, Instantaneous)" : spsPower3phInstantaneousLib/Power (3ph, Instantaneous)
  Product : Product
  Product1 : Product
  Product2 : Product
  Rate Limiter : RateLimiter  RisingSlewLimit=5  FallingSlewLimit=-5  SampleTimeMode=inherited
  Scope : Scope
      settings: ActiveDisplayYMinimum=-423.55092  ActiveDisplayYMaximum=423.50002  DataLoggingVariableName=ScopeData3
  Scope1 : Scope  NumInputPorts=4
      settings: ActiveDisplayYMinimum=-435.11495  ActiveDisplayYMaximum=432.79484  DataLoggingVariableName=ScopeData5
  Scope4 : Scope  NumInputPorts=2
      settings: ActiveDisplayYMinimum=-1.88604  ActiveDisplayYMaximum=1.48102  DataLoggingVariableName=ScopeData8
  Selector : Selector  InputPortWidth=3  IndexOptions=Index vector (dialog)  Indices=[2]  OutputSizes=1
  Step : Step  Time=0  After=0.5  SampleTime=0
  Sum37 : Sum  Inputs=|+-
  Terminator : Terminator
  Terminator1 : Terminator
  Three-Phase V-I Measurement1 : spsThreePhaseVIMeasurementLib/Three-Phase V-I Measurement  VoltageMeasurement=no  SetLabelV=off  LabelV=Vabc  Vpu=off  VpuLL=off  CurrentMeasurement=yes  SetLabelI=off  LabelI=Iabc  Ipu=off  Pbase=100e6  Vbase=500e3  OutputType=Complex  PhasorSimulation=off  PSBequivalent=0
  Three-Phase V-I Measurement2 : spsThreePhaseVIMeasurementLib/Three-Phase V-I Measurement  VoltageMeasurement=phase-to-phase  SetLabelV=off  LabelV=Vabc  Vpu=off  VpuLL=off  CurrentMeasurement=yes  SetLabelI=off  LabelI=Iabc  Ipu=off  Pbase=100e6  Vbase=500e3  OutputType=Complex  PhasorSimulation=off  PSBequivalent=0
  Unit Delay : UnitDelay  SampleTime=1/fsw1
  VSC : Subsystem
  Zero-Order Hold2 : ZeroOrderHold  SampleTime=1/fsw1
  Zero-Order Hold3 : ZeroOrderHold  SampleTime=1/fsw1
  Zero-Order Hold4 : ZeroOrderHold  SampleTime=1/fsw1
  abc to dq0 : spsabctodq0Lib/abc to dq0  Alignment=90 degrees behind phase A axis
  abc to dq2 : spsabctodq0Lib/abc to dq0  Alignment=90 degrees behind phase A axis
  abc to dq3 : spsabctodq0Lib/abc to dq0  Alignment=90 degrees behind phase A axis
  dq0 to abc2 : spsdq0toabcLib/dq0 to abc  Alignment=90 degrees behind phase A axis
  a : PMIOPort  Side=Right
  b : PMIOPort  Port=2  Side=Right
  c : PMIOPort  Port=3  Side=Right
  wires:
  [Vpcc] -> Gain9/1
  Three-Phase V-I Measurement2/1 -> Zero-Order Hold3/1
  [Vline] -> Line to Phase/1(In1)
  Line to Phase/1(Out1) -> [Vpcc]
  Constant45/1 -> Mux9/2
  dq0 to abc2/1 -> Gain6/1
  Zero-Order Hold2/1 -> [Iabc]
  Three-Phase V-I Measurement1/1 -> Zero-Order Hold2/1
  Demux3/3 -> Terminator/1
  Zero-Order Hold4/1 -> [Ipcc]
  [theta] -> dq0 to abc2/2
  Demux1/2 -> [Iq]
  Gain6/1 -> Unit Delay/1
  abc to dq3/1 -> Demux3/1
  Demux3/1 -> [Vd]
  [Id] -> Mux2/1
  Mux2/1 -> Scope4/2, Sum37/2
  [Iq] -> Mux2/2
  Mux9/1 -> dq0 to abc2/1
  Constant55/1 -> Mux3/2
  [Iabc] -> Gain10/1
  Demux3/2 -> [Vq]
  Demux1/3 -> Terminator1/1
  Gain9/1 -> abc to dq3/1
  Demux1/1 -> [Id]
  Zero-Order Hold3/1 -> [Vline]
  Unit Delay/1 -> Scope/1, [ref]
  [ref] -> VSC/1(Uabcref)
  Three-Phase V-I Measurement2/2 -> Zero-Order Hold4/1
  Gain10/1 -> abc to dq0/1
  [theta] -> abc to dq3/2
  Mux3/1 -> Scope4/1, Sum37/1
  [theta] -> abc to dq0/2
  abc to dq0/1 -> Demux1/1
  Discrete-Time Integrator2/1 -> [theta], abc to dq2/2
  Constant1/1 -> Add1/1
  PID/1(Out1) -> Add1/2
  Add1/1 -> Gain1/1
  abc to dq2/1 -> Selector/1
  PID Controller1/1 -> Mux9/1
  Gain2/1 -> abc to dq2/1
  [Vpcc] -> Gain2/1
  "Power (3ph, Instantaneous)"/1 -> Gain/1
  "Power (3ph, Instantaneous)"/2 -> Gain5/1
  [Ipcc] -> "Power (3ph, Instantaneous)"/2
  [Vpcc] -> "Power (3ph, Instantaneous)"/1
  Gain/1 -> [P], Mux1/1
  [Vpcc] -> Scope1/1
  Gain5/1 -> [Q], Mux1/2
  [PQ] -> Scope1/3
  [Ipcc] -> Scope1/2
  [omga] -> Scope1/4
  Mux1/1 -> [PQ]
  Sum37/1 -> Product/1
  [RST] -> Product/2
  Product/1 -> PID Controller1/1
  Selector/1 -> Product1/2
  Product1/1 -> PID/1(In1)
  Product2/1 -> Discrete-Time Integrator2/1
  Gain1/1 -> [omga], Product2/1
  Constant/1 -> Product1/1
  Constant2/1 -> Product2/2
  Rate Limiter/1 -> Mux3/1
  Step/1 -> Rate Limiter/1
  Constant4/1 -> [RST]
  connections:
  Load2/RConn1 -- Load2/RConn3 -- Load2/RConn2
  LCL-Inverter2/RConn3 -- Load2/LConn3 -- Three-Phase V-I Measurement2/LConn3
  LCL-Inverter2/RConn2 -- Load2/LConn2 -- Three-Phase V-I Measurement2/LConn2
  LCL-Inverter2/RConn1 -- Load2/LConn1 -- Three-Phase V-I Measurement2/LConn1
  LCL-Inverter3/LConn2 -- Three-Phase V-I Measurement2/RConn2
  LCL-Inverter3/LConn3 -- Three-Phase V-I Measurement2/RConn3
  Three-Phase V-I Measurement1/LConn1 -- VSC/RConn1
  LCL-Inverter3/RConn3 -- c/RConn1
  Three-Phase V-I Measurement1/RConn3 -- LCL-Inverter2/LConn3
  Three-Phase V-I Measurement1/RConn2 -- LCL-Inverter2/LConn2
  Three-Phase V-I Measurement1/RConn1 -- LCL-Inverter2/LConn1
  Three-Phase V-I Measurement1/LConn2 -- VSC/RConn2
  LCL-Inverter3/RConn1 -- a/RConn1
  LCL-Inverter3/LConn1 -- Three-Phase V-I Measurement2/RConn1
  Three-Phase V-I Measurement1/LConn3 -- VSC/RConn3
  LCL-Inverter3/RConn2 -- b/RConn1

== system Microgrid_LCTLM_server/Subsystem/LOAD1 ==
  Constant8 : Constant  Value=0
  Rload1 : spsThreePhaseSeriesRLCBranchLib/Three-Phase Series RLC Branch  LConnTagsString=A|B|C  RConnTagsString=A|B|C  BranchType=R  Resistance=Rload1  Inductance=Lline1  Capacitance=1e-6  Measurements=None
  Three-Phase Breaker3 : spsThreePhaseBreakerLib/Three-Phase Breaker  InitialState=open  SwitchA=on  SwitchB=on  SwitchC=on  SwitchTimes=1.5  External=on  BreakerResistance=Rbreaker  SnubberResistance=1e6  SnubberCapacitance=inf  Measurements=None
  A : PMIOPort  Side=Left
  B : PMIOPort  Port=2  Side=Left
  C : PMIOPort  Port=3  Side=Left
  wires:
  Constant8/1 -> Three-Phase Breaker3/1
  connections:
  A/RConn1 -- Three-Phase Breaker3/LConn1
  Three-Phase Breaker3/RConn3 -- Rload1/LConn3
  B/RConn1 -- Three-Phase Breaker3/LConn2
  Rload1/RConn2 -- Rload1/RConn1 -- Rload1/RConn3
  Three-Phase Breaker3/RConn1 -- Rload1/LConn1
  Three-Phase Breaker3/RConn2 -- Rload1/LConn2
  C/RConn1 -- Three-Phase Breaker3/LConn3

== system Microgrid_LCTLM_server/Subsystem/LOAD3 ==
  Constant14 : Constant  Value=0
  Rload3 : spsThreePhaseSeriesRLCBranchLib/Three-Phase Series RLC Branch  LConnTagsString=A|B|C  RConnTagsString=A|B|C  BranchType=R  Resistance=Rload3  Inductance=Lline1  Capacitance=1e-6  Measurements=None
  Three-Phase Breaker2 : spsThreePhaseBreakerLib/Three-Phase Breaker  InitialState=open  SwitchA=on  SwitchB=on  SwitchC=on  SwitchTimes=1.5  External=on  BreakerResistance=Rbreaker  SnubberResistance=1e6  SnubberCapacitance=inf  Measurements=None
  A : PMIOPort  Side=Left
  B : PMIOPort  Port=2  Side=Left
  C : PMIOPort  Port=3  Side=Left
  wires:
  Constant14/1 -> Three-Phase Breaker2/1
  connections:
  Three-Phase Breaker2/LConn2 -- B/RConn1
  Three-Phase Breaker2/RConn1 -- Rload3/LConn1
  Three-Phase Breaker2/RConn3 -- Rload3/LConn3
  Rload3/RConn3 -- Rload3/RConn1 -- Rload3/RConn2
  Three-Phase Breaker2/RConn2 -- Rload3/LConn2
  Three-Phase Breaker2/LConn1 -- A/RConn1
  Three-Phase Breaker2/LConn3 -- C/RConn1

== system Microgrid_LCTLM_server/Subsystem/LOAD4 ==
  Constant1 : Constant
  Rload2 : spsThreePhaseSeriesRLCBranchLib/Three-Phase Series RLC Branch  LConnTagsString=A|B|C  RConnTagsString=A|B|C  BranchType=R  Resistance=Rload2  Inductance=Lline1  Capacitance=1e-6  Measurements=None
  Three-Phase Breaker1 : spsThreePhaseBreakerLib/Three-Phase Breaker  InitialState=open  SwitchA=on  SwitchB=on  SwitchC=on  SwitchTimes=1.5  External=on  BreakerResistance=Rbreaker  SnubberResistance=1e6  SnubberCapacitance=inf  Measurements=None
  A : PMIOPort  Side=Left
  B : PMIOPort  Port=2  Side=Left
  C : PMIOPort  Port=3  Side=Left
  wires:
  Constant1/1 -> Three-Phase Breaker1/1
  connections:
  Three-Phase Breaker1/RConn3 -- Rload2/LConn3
  B/RConn1 -- Three-Phase Breaker1/LConn2
  Three-Phase Breaker1/RConn1 -- Rload2/LConn1
  C/RConn1 -- Three-Phase Breaker1/LConn3
  Rload2/RConn3 -- Rload2/RConn2 -- Rload2/RConn1
  Three-Phase Breaker1/RConn2 -- Rload2/LConn2
  A/RConn1 -- Three-Phase Breaker1/LConn1

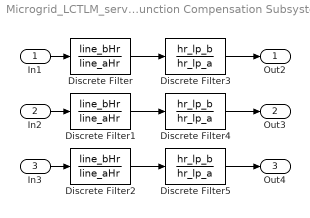
== system Microgrid_LCTLM_server/Subsystem/Propagation Function Compensation Subsystem ==
  In1 : Inport
  In2 : Inport  Port=2
  In3 : Inport  Port=3
  Discrete Filter : DiscreteFilter  LoadFcn=dspblkCoreblockFVToolHelper(gcbh,'load');  Numerator=line_bHr  Denominator=line_aHr
      settings: CopyFcn=dspblkCoreblockFVToolHelper(gcbh,'copy');  DeleteFcn=dspblkCoreblockFVToolHelper(gcbh,'close');  ModelCloseFcn=dspblkCoreblockFVToolHelper(gcbh,'close');  PreSaveFcn=dspblkCoreblockFVToolHelper(gcbh,'presave');  PostSaveFcn=dspblkCoreblockFVToolHelper(gcbh,'postsave');  CloseFcn=dspblkCoreblockFVToolHelper(gcbh,'close');
  Discrete Filter1 : DiscreteFilter  LoadFcn=dspblkCoreblockFVToolHelper(gcbh,'load');  Numerator=line_bHr  Denominator=line_aHr
      settings: CopyFcn=dspblkCoreblockFVToolHelper(gcbh,'copy');  DeleteFcn=dspblkCoreblockFVToolHelper(gcbh,'close');  ModelCloseFcn=dspblkCoreblockFVToolHelper(gcbh,'close');  PreSaveFcn=dspblkCoreblockFVToolHelper(gcbh,'presave');  PostSaveFcn=dspblkCoreblockFVToolHelper(gcbh,'postsave');  CloseFcn=dspblkCoreblockFVToolHelper(gcbh,'close');
  Discrete Filter2 : DiscreteFilter  LoadFcn=dspblkCoreblockFVToolHelper(gcbh,'load');  Numerator=line_bHr  Denominator=line_aHr
      settings: CopyFcn=dspblkCoreblockFVToolHelper(gcbh,'copy');  DeleteFcn=dspblkCoreblockFVToolHelper(gcbh,'close');  ModelCloseFcn=dspblkCoreblockFVToolHelper(gcbh,'close');  PreSaveFcn=dspblkCoreblockFVToolHelper(gcbh,'presave');  PostSaveFcn=dspblkCoreblockFVToolHelper(gcbh,'postsave');  CloseFcn=dspblkCoreblockFVToolHelper(gcbh,'close');
  Discrete Filter3 : DiscreteFilter  LoadFcn=dspblkCoreblockFVToolHelper(gcbh,'load');  Numerator=hr_lp_b  Denominator=hr_lp_a
      settings: CopyFcn=dspblkCoreblockFVToolHelper(gcbh,'copy');  DeleteFcn=dspblkCoreblockFVToolHelper(gcbh,'close');  ModelCloseFcn=dspblkCoreblockFVToolHelper(gcbh,'close');  PreSaveFcn=dspblkCoreblockFVToolHelper(gcbh,'presave');  PostSaveFcn=dspblkCoreblockFVToolHelper(gcbh,'postsave');  CloseFcn=dspblkCoreblockFVToolHelper(gcbh,'close');
  Discrete Filter4 : DiscreteFilter  LoadFcn=dspblkCoreblockFVToolHelper(gcbh,'load');  Numerator=hr_lp_b  Denominator=hr_lp_a
      settings: CopyFcn=dspblkCoreblockFVToolHelper(gcbh,'copy');  DeleteFcn=dspblkCoreblockFVToolHelper(gcbh,'close');  ModelCloseFcn=dspblkCoreblockFVToolHelper(gcbh,'close');  PreSaveFcn=dspblkCoreblockFVToolHelper(gcbh,'presave');  PostSaveFcn=dspblkCoreblockFVToolHelper(gcbh,'postsave');  CloseFcn=dspblkCoreblockFVToolHelper(gcbh,'close');
  Discrete Filter5 : DiscreteFilter  LoadFcn=dspblkCoreblockFVToolHelper(gcbh,'load');  Numerator=hr_lp_b  Denominator=hr_lp_a
      settings: CopyFcn=dspblkCoreblockFVToolHelper(gcbh,'copy');  DeleteFcn=dspblkCoreblockFVToolHelper(gcbh,'close');  ModelCloseFcn=dspblkCoreblockFVToolHelper(gcbh,'close');  PreSaveFcn=dspblkCoreblockFVToolHelper(gcbh,'presave');  PostSaveFcn=dspblkCoreblockFVToolHelper(gcbh,'postsave');  CloseFcn=dspblkCoreblockFVToolHelper(gcbh,'close');
  Out2 : Outport
  Out3 : Outport  Port=2
  Out4 : Outport  Port=3
  wires:
  In1/1 -> Discrete Filter/1
  In2/1 -> Discrete Filter1/1
  In3/1 -> Discrete Filter2/1
  Discrete Filter/1 -> Discrete Filter3/1
  Discrete Filter3/1 -> Out2/1
  Discrete Filter1/1 -> Discrete Filter4/1
  Discrete Filter4/1 -> Out3/1
  Discrete Filter5/1 -> Out4/1
  Discrete Filter2/1 -> Discrete Filter5/1

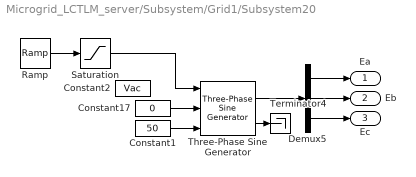
== system Microgrid_LCTLM_server/Subsystem/Grid1/Subsystem20 ==
  Constant1 : Constant  Value=50
  Constant17 : Constant  Value=0
  Constant2 : Constant  Value=Vac
  Demux5 : Demux  Outputs=3
  Ramp : simulink/Sources/Ramp  slope=Vac/0.01  start=0  InitialOutput=0
  Saturation : Saturate  UpperLimit=Vac  LowerLimit=0
  Terminator4 : Terminator
  Three-Phase Sine Generator : spsThreePhaseSineGeneratorLib/Three-Phase Sine Generator  Ts=1e-6
      settings: LibrarySourceBlock=|
      | sps_lib/Sources/Signal Generator Sources/Three-Phase
      | Sine Generator
  Ea : Outport
  Eb : Outport  Port=2
  Ec : Outport  Port=3
  wires:
  Three-Phase Sine Generator/1 -> Demux5/1
  Three-Phase Sine Generator/2 -> Terminator4/1
  Demux5/1 -> Ea/1
  Demux5/2 -> Eb/1
  Demux5/3 -> Ec/1
  Constant17/1 -> Three-Phase Sine Generator/2
  Constant1/1 -> Three-Phase Sine Generator/3
  Ramp/1 -> Saturation/1
  Saturation/1 -> Three-Phase Sine Generator/1

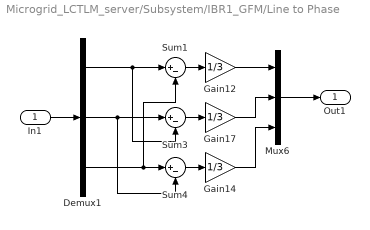
== system Microgrid_LCTLM_server/Subsystem/IBR1_GFM/Line to Phase ==
  In1 : Inport
  Demux1 : Demux  Outputs=3
  Gain12 : Gain  Gain=1/3
  Gain14 : Gain  Gain=1/3
  Gain17 : Gain  Gain=1/3
  Mux6 : Mux  Inputs=3
  Sum1 : Sum  Inputs=|+-
  Sum3 : Sum  Inputs=|+-
  Sum4 : Sum  Inputs=|+-
  Out1 : Outport
  wires:
  Sum3/1 -> Gain17/1
  Gain17/1 -> Mux6/2
  In1/1 -> Demux1/1
  Gain14/1 -> Mux6/3
  Sum1/1 -> Gain12/1
  Sum4/1 -> Gain14/1
  Demux1/3 -> Sum4/1, Sum1/2
  Demux1/2 -> Sum4/2, Sum3/1
  Gain12/1 -> Mux6/1
  Mux6/1 -> Out1/1
  Demux1/1 -> Sum3/2, Sum1/1
